simulink model "Partial_Response"  (Simulink 8.6)
settings: Solver=FixedStepDiscrete  StartTime=0  StopTime=inf  RelTol=1e-3
undefined symbols (not defined in the file or in its folder): dfilt, gcbh, magnitude, rcfiltgaincompat
libraries: commfilt2 x12, dspobslib x2, dspstat3 x2, simulink x2, commdigbbndam3 x1, commchan3 x1, dspsigops x1, commrandsrc2 x1
CloseFcn:
  | rtwprivate ssgencode ModelCloseRequest Nyquist_Bedingungen
settings Model: Creator=schwall  LastModifiedBy=wunsch
settings DataIOCC: SaveOutput=off  SignalLogging=off  SaveTime=off
settings DebuggingCC: FcnCallInpInsideContextMsg=UseLocalSettings

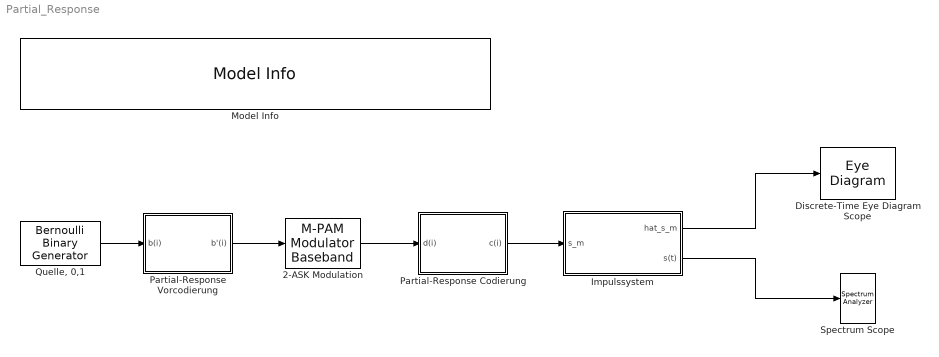
== system Partial_Response ==
  2-ASK Modulation : commdigbbndam3/M-PAM Modulator Baseband  M=2  InType=Bit  Enc=Binary  PowType=Average Power  MinDist=2  AvgPow=1  PeakPow=1  outDtype=double  outWordLen=16  outUDDataType=sfix(16)  outFracLenMode=Best precision  outFracLen=15
  Discrete-Time Eye Diagram Scope : EyeDiagram  Tag=EyeDiagram
  Impulssystem : Subsystem  mask(Impulssystem){rolloff_set=RRC Rolloff-Faktor 0, EsN0=100, abtast_set=0}
      mask prompts: rolloff_set "Impulsformung:"; EsN0 "Es/N0 [dB]:"; abtast_set "Abtastfehler (0...7)"
      mask help:
      | Kettenschaltung aus: Sendefilter -> Kanal -> AWGN -> Jitter -> Matched-Filter.
      | Interpolationsfaktor Sendefilter: I=8.
      mask TypeOptions rolloff_set: RRC Rolloff-Faktor 0 | RRC Rolloff-Faktor 0.2 | RRC Rolloff-Faktor 0.4 | RRC Rolloff-Faktor 0.6 | RRC Rolloff-Faktor 0.8 | RRC Rolloff-Faktor 1 | Rechteck-Filter
  Model Info : simulink/Model-Wide Utilities/Model Info  BlockCM=None  Frame=on  DisplayStringWithTags=|  HorizontalTextAlignment=Left  LeftAlignmentValue=0.02  SourceBlockDiagram=Partial_Response  TagMaxNumber=20
      | Demo Kontrollierte Intersymbolinterferenz - Partial-Response - Duobinaer-Code
      | Vorlesung Nachrichtentechnik II
      | Institut fuer Nachrichtentechnik (CEL)
  Partial-Response Codierung : Subsystem  mask(Partial-Response Codierung){prc_on_off=off}
      mask prompts: prc_on_off "Partial-Response Codierung"
      mask help:
      | Duobinaer-Codierung.
      | a_0=a_1=1
  Partial-Response Vorcodierung : Subsystem  mask(Partial-Response Vorcodierung){prv_on_off=off}
      mask prompts: prv_on_off "Duobinaer-Vorcodierung"
      mask help:
      | Duobinaer-Vorcodierung.
      | b_0=b_1=1
  "Quelle, 0,1" : commrandsrc2/Bernoulli Binary Generator  P=0.5  seed=61  Ts=1/100  frameBased=off  sampPerFrame=8  orient=off  outDataType=int32
  Spectrum Scope : SpectrumAnalyzer
  wires:
  Impulssystem/1(hat_s_m) -> Discrete-Time Eye Diagram Scope/1
  Partial-Response Codierung/1(c(i)) -> Impulssystem/1(s_m)
  "Quelle, 0,1"/1 -> Partial-Response Vorcodierung/1(b(i))
  Partial-Response Vorcodierung/1(b'(i)) -> 2-ASK Modulation/1
  2-ASK Modulation/1 -> Partial-Response Codierung/1(d(i))
  Impulssystem/2(s(t)) -> Spectrum Scope/1

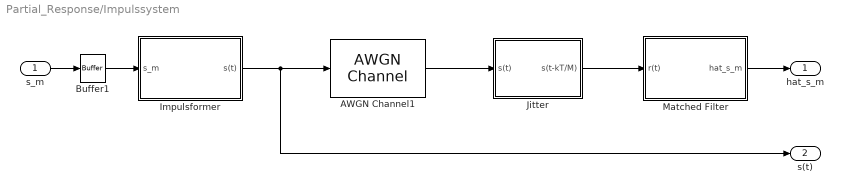
== system Partial_Response/Impulssystem ==
  s_m : Inport
  AWGN Channel1 : commchan3/AWGN Channel  InputProcessing=Columns as channels (frame based)  seed=67  noiseMode="Signal to noise ratio  (Es/No)"  EbNodB=EsN0  EsNodB=EsN0  SNRdB=10  bitsPerSym=1  Ps=1/8  Tsym=1/100  variance=1
  Buffer1 : Buffer  N=8  TreatMby1Signals=One channel  OutputFrames=off
  Impulsformer : Subsystem
  Jitter : Subsystem
  Matched Filter : Subsystem
  hat_s_m : Outport
  s(t) : Outport  Port=2
  wires:
  Impulsformer/1(s(t)) -> AWGN Channel1/1, s(t)/1
  AWGN Channel1/1 -> Jitter/1(s(t))
  Jitter/1(s(t-kT/M)) -> Matched Filter/1(r(t))
  s_m/1 -> Buffer1/1
  Matched Filter/1(hat_s_m) -> hat_s_m/1
  Buffer1/1 -> Impulsformer/1(s_m)

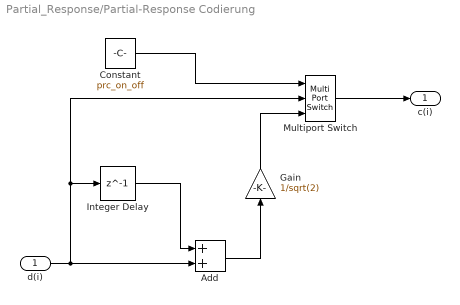
== system Partial_Response/Partial-Response Codierung ==
  d(i) : Inport
  Add : Sum
  Constant : Constant  Value=prc_on_off
  Gain : Gain  Gain=1/sqrt(2)
  Integer Delay : Delay  DelayLength=1  InputProcessing=Inherited
  Multiport Switch : MultiPortSwitch  DataPortOrder=Zero-based contiguous  Inputs=2  zeroidx=on
  c(i) : Outport
  wires:
  Integer Delay/1 -> Add/1
  d(i)/1 -> Add/2, Integer Delay/1, Multiport Switch/2
  Constant/1 -> Multiport Switch/1
  Multiport Switch/1 -> c(i)/1
  Add/1 -> Gain/1
  Gain/1 -> Multiport Switch/3

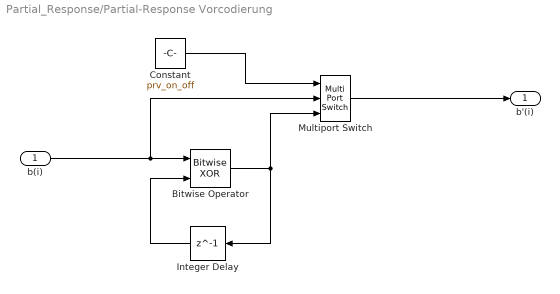
== system Partial_Response/Partial-Response Vorcodierung ==
  b(i) : Inport
  Bitwise Operator : simulink/Logic and Bit Operations/Bitwise Operator  logicop=XOR  UseBitMask=off  NumInputPorts=2  BitMask=bin2dec('11011001')  BitMaskRealWorld=Stored Integer
  Constant : Constant  Value=prv_on_off
  Integer Delay : Delay  DelayLength=1  InputProcessing=Inherited
  Multiport Switch : MultiPortSwitch  DataPortOrder=Zero-based contiguous  Inputs=2  zeroidx=on
  b'(i) : Outport
  wires:
  Bitwise Operator/1 -> Integer Delay/1, Multiport Switch/3
  Integer Delay/1 -> Bitwise Operator/2
  b(i)/1 -> Multiport Switch/2, Bitwise Operator/1
  Multiport Switch/1 -> b'(i)/1
  Constant/1 -> Multiport Switch/1

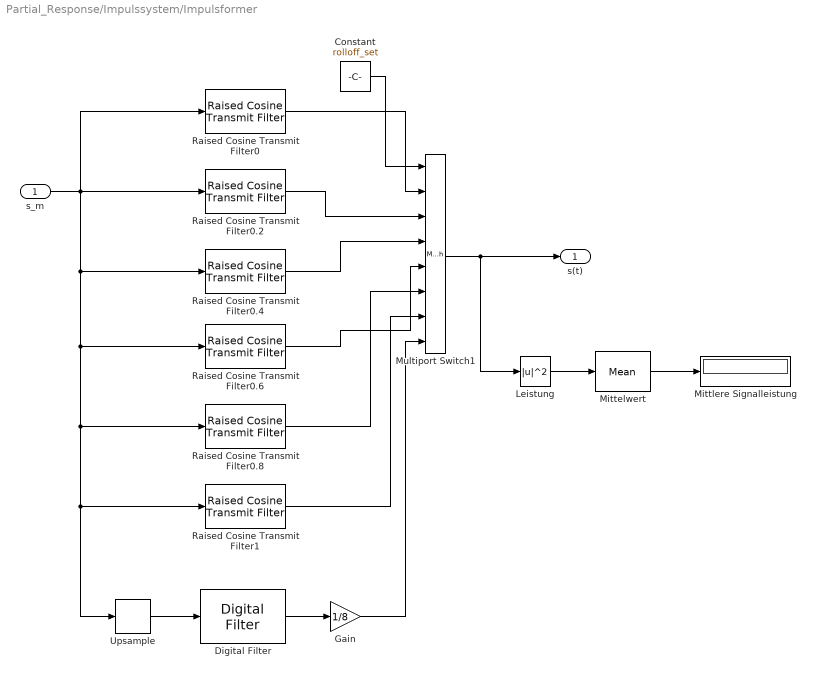
== system Partial_Response/Impulssystem/Impulsformer ==
  s_m : Inport
  Constant : Constant  Value=rolloff_set
  Digital Filter : dspobslib/Digital Filter  TypePopup=FIR (all zeros)  IIRFiltStruct=Direct form II transposed  AllPoleFiltStruct=Direct form  FIRFiltStruct=Direct form  CoeffSource=Specify via dialog  NumCoeffs=ones(8,1)  DenCoeffs=[1 0.1]  BiQuadCoeffs=[1 0.3 0.4 1 0.1 0.2]  LatticeCoeffs=[0.2 0.4]  denIgnore=on  FiltPerSampPopup=One filter per frame  IC=0  ICnum=0  ICden=0  roundingMode=Floor  overflowMode=off  ScaleValues=1  scaleValueFracLength=14  stageInFracLength=15  stageOutFracLength=15  FilterSource=Specify via dialog  dfiltObjectName=dfilt.dffir([1 2 1])  InputProcessing=Columns as channels (frame based)
  Gain : Gain  Gain=1/8
  Leistung : Math  Operator=magnitude^2  SaturateOnIntegerOverflow=on
  Mittelwert : dspstat3/Mean  run=on  reset_popup=None  InputProcessing=Columns as channels (frame based)  directionMode=Each column  dimension=1  roiEnable=off  roiType=Rectangles  roiPortion=Entire ROI  roiOutput=Individual statistics for each ROI  roiFlag=off  outputDataTypeStr=Inherit: Same as accumulator  outputLastDataTypeStr=Inherit: Same as accumulator  outputMin=[]  outputMax=[]  roundingMode=Floor  overflowMode=off
  Mittlere Signalleistung : Display
  Multiport Switch1 : MultiPortSwitch  Inputs=7
  Raised Cosine Transmit Filter0 : commfilt2/Raised Cosine Transmit Filter  filtType=Square root  filtSpan=2*(4)  currentFiltSpan=2*(4)  D=4  R=0  sampMode=Mute  saveAsFlag=0  N=8  framing=Maintain input frame rate  InputProcessing=Columns as channels (frame based)  checkGain=Normalized  filterGain=rcfiltgaincompat(gcbh)  checkCoeff=off  variableName=rcTxFilt  launchFVT=off  roundingMode=Floor  overflowMode=off
  Raised Cosine Transmit Filter0.2 : commfilt2/Raised Cosine Transmit Filter  filtType=Square root  filtSpan=2*(4)  currentFiltSpan=2*(4)  D=4  R=0.2  sampMode=Mute  saveAsFlag=0  N=8  framing=Maintain input frame rate  InputProcessing=Columns as channels (frame based)  checkGain=Normalized  filterGain=rcfiltgaincompat(gcbh)  checkCoeff=off  variableName=rcTxFilt1  launchFVT=off  roundingMode=Floor  overflowMode=off
  Raised Cosine Transmit Filter0.4 : commfilt2/Raised Cosine Transmit Filter  filtType=Square root  filtSpan=2*(4)  currentFiltSpan=2*(4)  D=4  R=0.4  sampMode=Mute  saveAsFlag=0  N=8  framing=Maintain input frame rate  InputProcessing=Columns as channels (frame based)  checkGain=Normalized  filterGain=rcfiltgaincompat(gcbh)  checkCoeff=off  variableName=rcTxFilt2  launchFVT=off  roundingMode=Floor  overflowMode=off
  Raised Cosine Transmit Filter0.6 : commfilt2/Raised Cosine Transmit Filter  filtType=Square root  filtSpan=2*(4)  currentFiltSpan=2*(4)  D=4  R=0.6  sampMode=Mute  saveAsFlag=0  N=8  framing=Maintain input frame rate  InputProcessing=Columns as channels (frame based)  checkGain=Normalized  filterGain=rcfiltgaincompat(gcbh)  checkCoeff=off  variableName=rcTxFilt3  launchFVT=off  roundingMode=Floor  overflowMode=off
  Raised Cosine Transmit Filter0.8 : commfilt2/Raised Cosine Transmit Filter  filtType=Square root  filtSpan=2*(4)  currentFiltSpan=2*(4)  D=4  R=0.8  sampMode=Mute  saveAsFlag=0  N=8  framing=Maintain input frame rate  InputProcessing=Columns as channels (frame based)  checkGain=Normalized  filterGain=rcfiltgaincompat(gcbh)  checkCoeff=off  variableName=rcTxFilt4  launchFVT=off  roundingMode=Floor  overflowMode=off
  Raised Cosine Transmit Filter1 : commfilt2/Raised Cosine Transmit Filter  filtType=Square root  filtSpan=2*(4)  currentFiltSpan=2*(4)  D=4  R=1  sampMode=Mute  saveAsFlag=0  N=8  framing=Maintain input frame rate  InputProcessing=Columns as channels (frame based)  checkGain=Normalized  filterGain=rcfiltgaincompat(gcbh)  checkCoeff=off  variableName=rcTxFilt5  launchFVT=off  roundingMode=Floor  overflowMode=off
  Upsample : dspsigops/Upsample  N=8  phase=0  InputProcessing=Columns as channels (frame based)  RateOptions=Enforce single-rate processing  ic=0  mode=Unused parameter value
  s(t) : Outport
  wires:
  s_m/1 -> Raised Cosine Transmit Filter0/1, Raised Cosine Transmit Filter0.2/1, Raised Cosine Transmit Filter0.4/1, Raised Cosine Transmit Filter0.8/1, Raised Cosine Transmit Filter1/1, Upsample/1, Raised Cosine Transmit Filter0.6/1
  Upsample/1 -> Digital Filter/1
  Mittelwert/1 -> Mittlere Signalleistung/1
  Leistung/1 -> Mittelwert/1
  Multiport Switch1/1 -> Leistung/1, s(t)/1
  Constant/1 -> Multiport Switch1/1
  Raised Cosine Transmit Filter0/1 -> Multiport Switch1/2
  Raised Cosine Transmit Filter0.2/1 -> Multiport Switch1/3
  Raised Cosine Transmit Filter0.4/1 -> Multiport Switch1/4
  Raised Cosine Transmit Filter0.6/1 -> Multiport Switch1/5
  Raised Cosine Transmit Filter0.8/1 -> Multiport Switch1/6
  Raised Cosine Transmit Filter1/1 -> Multiport Switch1/7
  Digital Filter/1 -> Gain/1
  Gain/1 -> Multiport Switch1/8

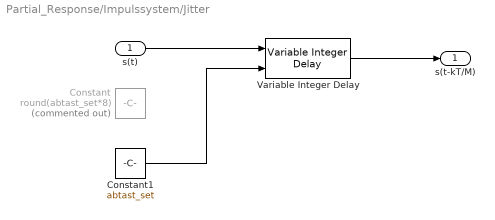
== system Partial_Response/Impulssystem/Jitter ==
  s(t) : Inport
  Constant : Constant  Commented=on  Value=round(abtast_set*8)
  Constant1 : Constant  Value=abtast_set
  Variable Integer Delay : dspobslib/Variable Integer Delay  dmax=64  InputProcessing=Columns as channels (frame based)  ic=0  noDFT=off
  s(t-kT/M) : Outport
  wires:
  Variable Integer Delay/1 -> s(t-kT/M)/1
  s(t)/1 -> Variable Integer Delay/1
  Constant1/1 -> Variable Integer Delay/2

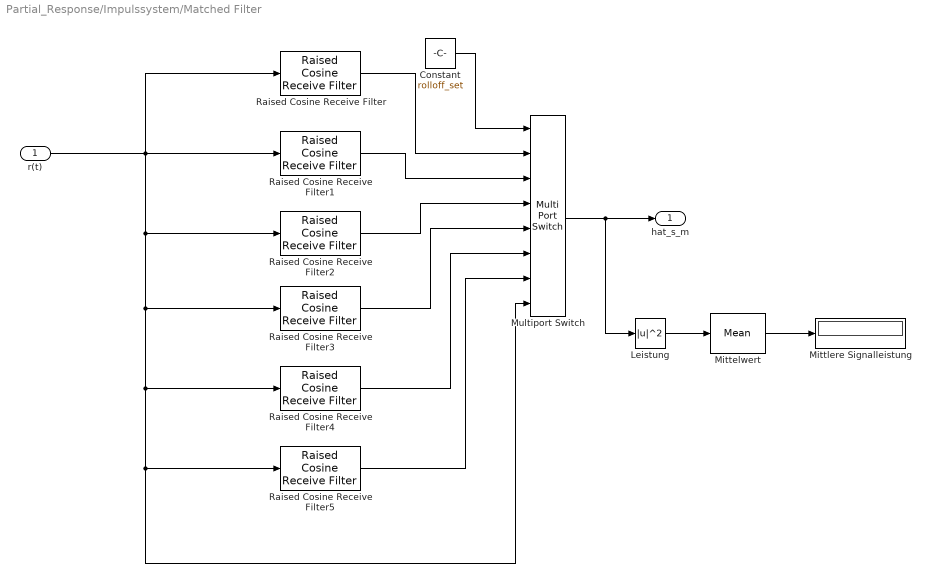
== system Partial_Response/Impulssystem/Matched Filter ==
  r(t) : Inport
  Constant : Constant  Value=rolloff_set
  Leistung : Math  Operator=magnitude^2  SaturateOnIntegerOverflow=on
  Mittelwert : dspstat3/Mean  run=on  reset_popup=None  InputProcessing=Columns as channels (frame based)  directionMode=Each column  dimension=1  roiEnable=off  roiType=Rectangles  roiPortion=Entire ROI  roiOutput=Individual statistics for each ROI  roiFlag=off  outputDataTypeStr=Inherit: Same as accumulator  outputLastDataTypeStr=Inherit: Same as accumulator  outputMin=[]  outputMax=[]  roundingMode=Floor  overflowMode=off
  Mittlere Signalleistung : Display
  Multiport Switch : MultiPortSwitch  Inputs=7
  Raised Cosine Receive Filter : commfilt2/Raised Cosine Receive Filter  filtType=Square root  N=8  filtSpan=2*(4)  currentFiltSpan=2*(4)  D=4  R=0  sampMode=Mute  saveAsFlag=0  rateMode=Downsampling  downFactor=1  downOffset=0  framing=Maintain input frame rate  InputProcessing=Columns as channels (frame based)  checkGain=Normalized  filterGain=rcfiltgaincompat(gcbh)  checkCoeff=off  variableName=rcRxFilt  launchFVT=off  roundingMode=Floor  overflowMode=off
  Raised Cosine Receive Filter1 : commfilt2/Raised Cosine Receive Filter  filtType=Square root  N=8  filtSpan=2*(4)  currentFiltSpan=2*(4)  D=4  R=0.2  sampMode=Mute  saveAsFlag=0  rateMode=Downsampling  downFactor=1  downOffset=0  framing=Maintain input frame rate  InputProcessing=Columns as channels (frame based)  checkGain=Normalized  filterGain=rcfiltgaincompat(gcbh)  checkCoeff=off  variableName=rcRxFilt1  launchFVT=off  roundingMode=Floor  overflowMode=off
  Raised Cosine Receive Filter2 : commfilt2/Raised Cosine Receive Filter  filtType=Square root  N=8  filtSpan=2*(4)  currentFiltSpan=2*(4)  D=4  R=0.4  sampMode=Mute  saveAsFlag=0  rateMode=Downsampling  downFactor=1  downOffset=0  framing=Maintain input frame rate  InputProcessing=Columns as channels (frame based)  checkGain=Normalized  filterGain=rcfiltgaincompat(gcbh)  checkCoeff=off  variableName=rcRxFilt2  launchFVT=off  roundingMode=Floor  overflowMode=off
  Raised Cosine Receive Filter3 : commfilt2/Raised Cosine Receive Filter  filtType=Square root  N=8  filtSpan=2*(4)  currentFiltSpan=2*(4)  D=4  R=0.6  sampMode=Mute  saveAsFlag=0  rateMode=Downsampling  downFactor=1  downOffset=0  framing=Maintain input frame rate  InputProcessing=Columns as channels (frame based)  checkGain=Normalized  filterGain=rcfiltgaincompat(gcbh)  checkCoeff=off  variableName=rcRxFilt3  launchFVT=off  roundingMode=Floor  overflowMode=off
  Raised Cosine Receive Filter4 : commfilt2/Raised Cosine Receive Filter  filtType=Square root  N=8  filtSpan=2*(4)  currentFiltSpan=2*(4)  D=4  R=0.8  sampMode=Mute  saveAsFlag=0  rateMode=Downsampling  downFactor=1  downOffset=0  framing=Maintain input frame rate  InputProcessing=Columns as channels (frame based)  checkGain=Normalized  filterGain=rcfiltgaincompat(gcbh)  checkCoeff=off  variableName=rcRxFilt4  launchFVT=off  roundingMode=Floor  overflowMode=off
  Raised Cosine Receive Filter5 : commfilt2/Raised Cosine Receive Filter  filtType=Square root  N=8  filtSpan=2*(4)  currentFiltSpan=2*(4)  D=4  R=1  sampMode=Mute  saveAsFlag=0  rateMode=Downsampling  downFactor=1  downOffset=0  framing=Maintain input frame rate  InputProcessing=Columns as channels (frame based)  checkGain=Normalized  filterGain=rcfiltgaincompat(gcbh)  checkCoeff=off  variableName=rcRxFilt5  launchFVT=off  roundingMode=Floor  overflowMode=off
  hat_s_m : Outport
  wires:
  Raised Cosine Receive Filter5/1 -> Multiport Switch/7
  Raised Cosine Receive Filter4/1 -> Multiport Switch/6
  Raised Cosine Receive Filter3/1 -> Multiport Switch/5
  Raised Cosine Receive Filter2/1 -> Multiport Switch/4
  Constant/1 -> Multiport Switch/1
  Multiport Switch/1 -> Leistung/1, hat_s_m/1
  Leistung/1 -> Mittelwert/1
  Mittelwert/1 -> Mittlere Signalleistung/1
  r(t)/1 -> Raised Cosine Receive Filter4/1, Raised Cosine Receive Filter5/1, Multiport Switch/8, Raised Cosine Receive Filter3/1, Raised Cosine Receive Filter2/1, Raised Cosine Receive Filter/1, Raised Cosine Receive Filter1/1
  Raised Cosine Receive Filter1/1 -> Multiport Switch/3
  Raised Cosine Receive Filter/1 -> Multiport Switch/2
